simulink model "pendulum"  (R2018a)
settings: Solver=ode45  StartTime=0.0  StopTime=10  RelTol=1e-3  EnableMultiTasking=on
values from neighbouring files (symbols this model uses):
  b = 4    [init.m]
  K1 = -15    [init.m]
  K2 = -1    [init.m]
  K3 = M1*l/(M2+M1)    (= 0.0909090909091)    [init.m]
  K4 = g/l    (= 9.8)    [init.m]
  K5 = 1/l    (= 1)    [init.m]
  Phi0 = -80    [init.m]
libraries: simulink_extras x1, aerolibanimutils x1
settings Model: Creator=Daddy  LastModifiedBy=D
settings DataIOCC: LimitDataPoints=on  SaveFormat=Array
settings OptimizationCC: LifeSpan=inf
settings DebuggingCC: SolverPrmCheckMsg=warning  SFUnexpectedBacktrackingDiag=warning  SFNoUnconditionalDefaultTransitionDiag=warning  SFExecutionAtInitializationDiag=none
settings HardwareCC: ProdBitPerPointer=32  ProdBitPerSizeT=32  ProdBitPerPtrDiffT=32  ProdLargestAtomicFloat=None  ProdIntDivRoundTo=Undefined  ProdEndianess=Unspecified  ProdWordSize=32  ProdHWDeviceType=32-bit Generic
settings ModelReferenceCC: PropagateSignalLabelsOutOfModel=off
settings CodeAppCC: StateflowObjectComments=on
settings GRTTargetCC: TargetLangStandard=C89/C90 (ANSI)  GeneratePreprocessorConditionals=Disable all
settings ConfigComp: CovMetricSettings=dw  CovHtmlReporting=on  CovSaveCumulativeToWorkspaceVar=on  CovSaveSingleToWorkspaceVar=on  CovExternalEMLEnable=off  CovSFcnEnable=off

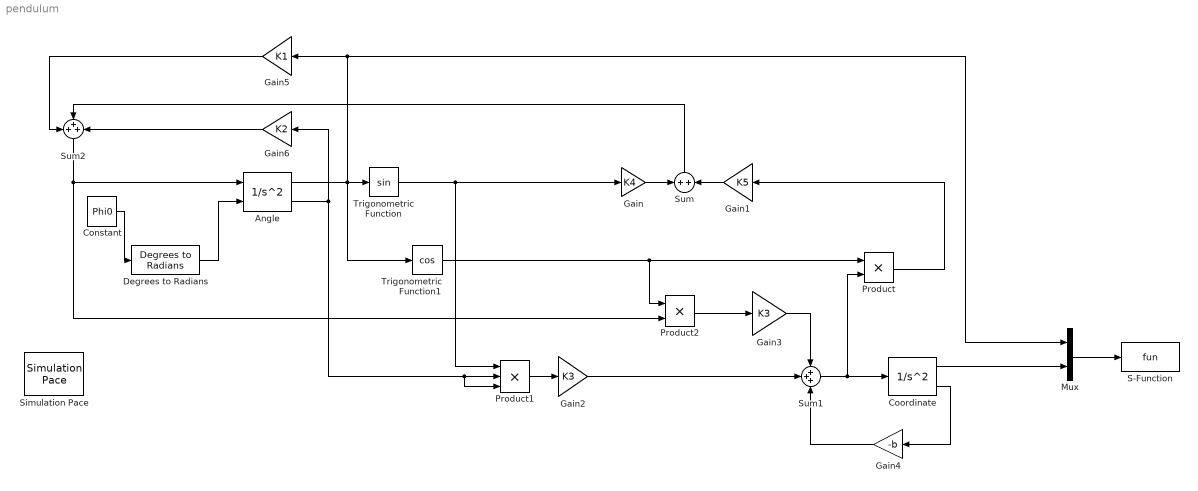
== system pendulum ==
  Angle : SecondOrderIntegrator  ICSourceX=external  ICX=2
  Constant : Constant  Value=Phi0
  Coordinate : SecondOrderIntegrator
  Degrees to Radians : simulink_extras/Transformations/Degrees to Radians
  Gain : Gain  Gain=K4
  Gain1 : Gain  Gain=K5  RndMeth=Round
  Gain2 : Gain  Gain=K3
  Gain3 : Gain  Gain=K3
  Gain4 : Gain  Gain=-b
  Gain5 : Gain  Gain=K1  RndMeth=Round
  Gain6 : Gain  Gain=K2
  Mux : Mux  Inputs=2
  Product : Product
  Product1 : Product  Inputs=3
  Product2 : Product
  S-Function : S-Function  FunctionName=fun  Parameters=4 5  SFunctionDeploymentMode=off  EnableBusSupport=off
  Simulation Pace : aerolibanimutils/Simulation Pace  SimulationPace=2  SleepMode=MATLAB Thread  OutputPaceError=off  SampleTime=1/30
      settings: AttributesFormatString=%<SimulationPace> sec/sec
  Sum : Sum  Inputs=+|+
  Sum1 : Sum  Inputs=+++
  Sum2 : Sum  Inputs=+++
  Trigonometric Function : Trigonometry
  Trigonometric Function1 : Trigonometry  Operator=cos
  wires:
  Angle/1 -> Trigonometric Function/1, Mux/1, Gain5/1, Trigonometric Function1/1
  Trigonometric Function/1 -> Gain/1, Product1/1
  Trigonometric Function1/1 -> Product/1, Product2/1
  Angle/2 -> Product1/3, Product1/2, Gain6/1
  Product1/1 -> Gain2/1
  Product2/1 -> Gain3/1
  Gain/1 -> Sum/1
  Coordinate/2 -> Gain4/1
  Gain4/1 -> Sum1/3
  Sum2/1 -> Product2/2, Angle/1
  Mux/1 -> S-Function/1
  Degrees to Radians/1 -> Angle/2
  Constant/1 -> Degrees to Radians/1
  Coordinate/1 -> Mux/2
  Sum1/1 -> Product/2, Coordinate/1
  Gain6/1 -> Sum2/3
  Product/1 -> Gain1/1
  Gain1/1 -> Sum/2
  Gain2/1 -> Sum1/2
  Gain3/1 -> Sum1/1
  Gain5/1 -> Sum2/1
  Sum/1 -> Sum2/2
